simulink model "Problem3"  (R2020b)
settings: Solver=VariableStepAuto  StartTime=0.0  StopTime=10.0  RelTol=1e-3
values from neighbouring files (symbols this model uses):
  a1 = -0.1584    [Problem3_Startup.m]
  b0 = 0.5792    [Problem3_Startup.m]
  b1 = -0.5792    [Problem3_Startup.m]
settings Model: Creator=Shirish  LastModifiedBy=Shirish

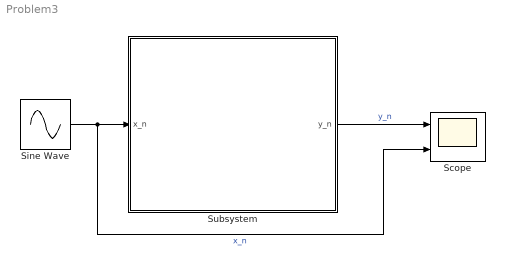
== system Problem3 ==
  Scope : Scope  NumInputPorts=2
  Sine Wave : Sin  Frequency=4500*pi*4  SampleTime=1/5000
  Subsystem : Subsystem
  wires:
  Sine Wave/1 -> Scope/2, Subsystem/1(x_n)  "x_n"
  Subsystem/1(y_n) -> Scope/1  "y_n"

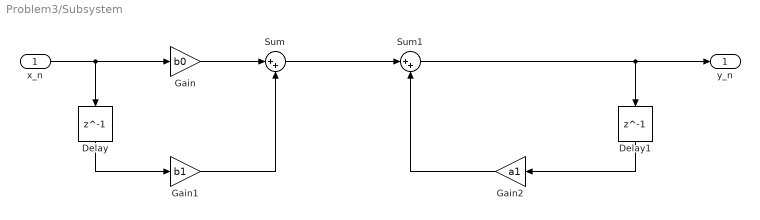
== system Problem3/Subsystem ==
  x_n : Inport
  Delay : Delay  DelayLength=1
  Delay1 : Delay  DelayLength=1
  Gain : Gain  Gain=b0
  Gain1 : Gain  Gain=b1
  Gain2 : Gain  Gain=a1
  Sum : Sum  Inputs=|++
  Sum1 : Sum  Inputs=|++
  y_n : Outport
  wires:
  Gain/1 -> Sum/1
  Sum1/1 -> y_n/1, Delay1/1
  Delay/1 -> Gain1/1
  Gain1/1 -> Sum/2
  Gain2/1 -> Sum1/2
  Sum/1 -> Sum1/1
  x_n/1 -> Gain/1, Delay/1
  Delay1/1 -> Gain2/1
